simulink model "s12_euler_ssprk3_periodic_ref"  (R2026a)
settings: Solver=FixedStepDiscrete  StopTime=0  FixedStep=1
model workspace (MAT data in the model file):
  S12_PRK3_BaseState = Simulink.Parameter
  S12_PRK3_BaseState.Value = [1.1  1.1  1.1  1.1  1.1  1.1  1.1  1.1; 0.22  0.22  0.22  0.22  0.22  0.22  0.22  0.22; 2.522  2.522  2.522  2.522  2.522  2.522  2.522  2.522]
  S12_PRK3_BaseState.Complexity = 'real'
  S12_PRK3_BaseState.Dimensions = [3 8]
  S12_PRK3_BaseState.DataType = 'auto'
  S12_PRK3_EulerState = Simulink.Parameter
  S12_PRK3_EulerState.Value = [1.1  1.1  1.1  1.1  1.1  1.1  1.1  1.1; 0.22  0.22  0.22  0.22  0.22  0.22  0.22  0.22; 2.522  2.522  2.522  2.522  2.522  2.522  2.522  2.522]
  S12_PRK3_EulerState.Complexity = 'real'
  S12_PRK3_EulerState.Dimensions = [3 8]
  S12_PRK3_EulerState.DataType = 'auto'
  S12_PRK3_StageIndex = Simulink.Parameter
  S12_PRK3_StageIndex.Value = 1
  S12_PRK3_StageIndex.Complexity = 'real'
  S12_PRK3_StageIndex.Dimensions = [1 1]
  S12_PRK3_StageIndex.DataType = 'auto'
settings Model: Creator=Jovi  LastModifiedBy=Jovi

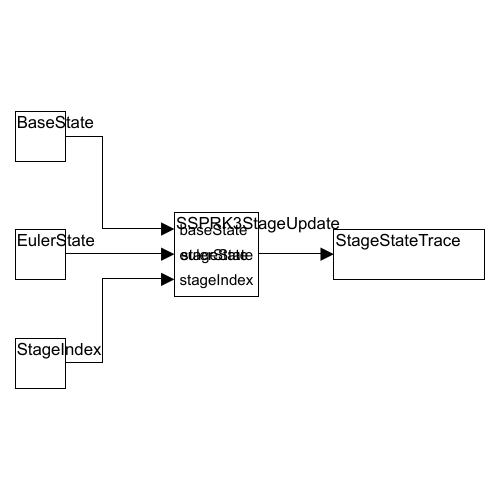
[thumbnail: Simulink's stored preview of the top-level diagram]
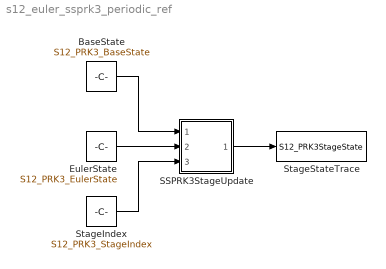
== system s12_euler_ssprk3_periodic_ref ==
  BaseState : Constant  Value=S12_PRK3_BaseState
  EulerState : Constant  Value=S12_PRK3_EulerState
  SSPRK3StageUpdate : MATLAB Function  TreatAsAtomicUnit=on
  StageIndex : Constant  Value=S12_PRK3_StageIndex
  StageStateTrace : ToWorkspace  VariableName=S12_PRK3StageState
  wires:
  SSPRK3StageUpdate/1(stageState) -> StageStateTrace/1
  StageIndex/1 -> SSPRK3StageUpdate/3(stageIndex)
  EulerState/1 -> SSPRK3StageUpdate/2(eulerState)
  BaseState/1 -> SSPRK3StageUpdate/1(baseState)

== matlab function s12_euler_ssprk3_periodic_ref/SSPRK3StageUpdate ==
  data: baseState input; stageState output; eulerState input; stageIndex input
function stageState = SSPRK3StageUpdate(baseState,eulerState,stageIndex)
%#codegen
if stageIndex == 1
    stageState = eulerState;
elseif stageIndex == 2
    stageState = 0.75*baseState + 0.25*eulerState;
elseif stageIndex == 3
    stageState = (1.0/3.0)*baseState + (2.0/3.0)*eulerState;
else
    error('S12:SSPRK3:InvalidStage','stageIndex must be 1, 2, or 3.');
end
end
